simulink library "time_coord_rotation_lib"  (R2016b)
settings: Solver=VariableStepAuto  StartTime=0.0  StopTime=10.0  RelTol=1e-3
undefined symbols (not defined in the file or in its folder): fsw_params
libraries: coord_rotation_lib x1, time_conversion_lib x1
settings Model: Creator=taylorreynolds  LastModifiedBy=taylorreynolds

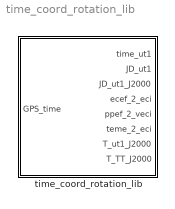
== system time_coord_rotation_lib ==
  time_coord_rotation_lib : Subsystem

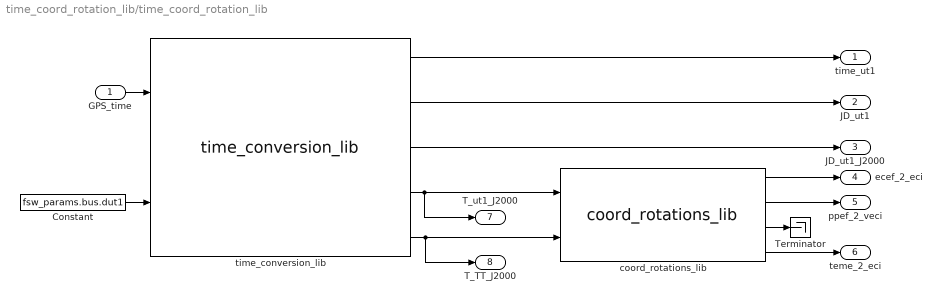
== system time_coord_rotation_lib/time_coord_rotation_lib ==
  GPS_time : Inport
  Constant : Constant  Value=fsw_params.bus.dut1
  Terminator : Terminator
  coord_rotations_lib : coord_rotation_lib/coord_rotations_lib
  time_conversion_lib : time_conversion_lib/time_conversion_lib
  time_ut1 : Outport
  JD_ut1 : Outport  Port=2
  JD_ut1_J2000 : Outport  Port=3
  ecef_2_eci : Outport  Port=4
  ppef_2_veci : Outport  Port=5
  teme_2_eci : Outport  Port=6
  T_ut1_J2000 : Outport  Port=7
  T_TT_J2000 : Outport  Port=8
  wires:
  GPS_time/1 -> time_conversion_lib/1
  Constant/1 -> time_conversion_lib/2
  time_conversion_lib/4 -> T_ut1_J2000/1, coord_rotations_lib/1
  time_conversion_lib/5 -> T_TT_J2000/1, coord_rotations_lib/2
  time_conversion_lib/1 -> time_ut1/1
  time_conversion_lib/2 -> JD_ut1/1
  time_conversion_lib/3 -> JD_ut1_J2000/1
  coord_rotations_lib/1 -> ecef_2_eci/1
  coord_rotations_lib/2 -> ppef_2_veci/1
  coord_rotations_lib/4 -> teme_2_eci/1
  coord_rotations_lib/3 -> Terminator/1
